simulink model "RPI1Deployment"  (R2026a)
settings: Solver=FixedStepDiscrete  StopTime=inf  FixedStep=rccar.SampleTime  EnableMultiTasking=on
InitFcn:
  | rccarRoot=fileparts(fileparts(fileparts(get_param(bdroot,'FileName')))); addpath(genpath(rccarRoot)); setupRCCarProject; clear rccarRoot;
undefined symbols (not defined in the file): rccar
libraries: raspberrypiNetworklib x3, simulink x1
settings Model: Creator=taegon  LastModifiedBy=taegon
settings SolverCC: PositivePriorityOrder=on
settings OptimizationCC: MaxStackSize=200000
settings HardwareCC: ProdBitPerLong=64.0  ProdLargestAtomicInteger=LongLong  ProdLargestAtomicFloat=Double  ProdHWDeviceType=ARM Compatible->ARM Cortex-A (64-bit)
settings RTWCC: SystemTargetFile=ert.tlc  HardwareBoard=Raspberry Pi (64bit)  TLCOptions="-aInlineSetEventsForThisBaseRateFcn=TLC_FALSE -aSuppressMultiTaskScheduler=TLC_FALSE  -aRateBasedStepFcn=0"  Toolchain=GNU GCC RPIUtils  BuildConfiguration=Faster Runs  Description=Embedded Coder
settings ERTTargetCC: ExtModeTransport=2.0  SupportVariableSizeSignals=on

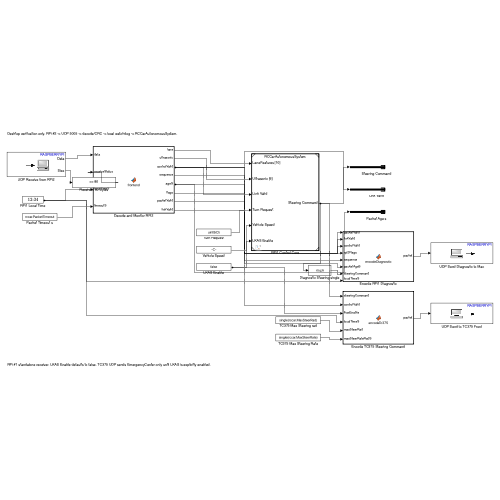
[thumbnail: Simulink's stored preview of the top-level diagram]
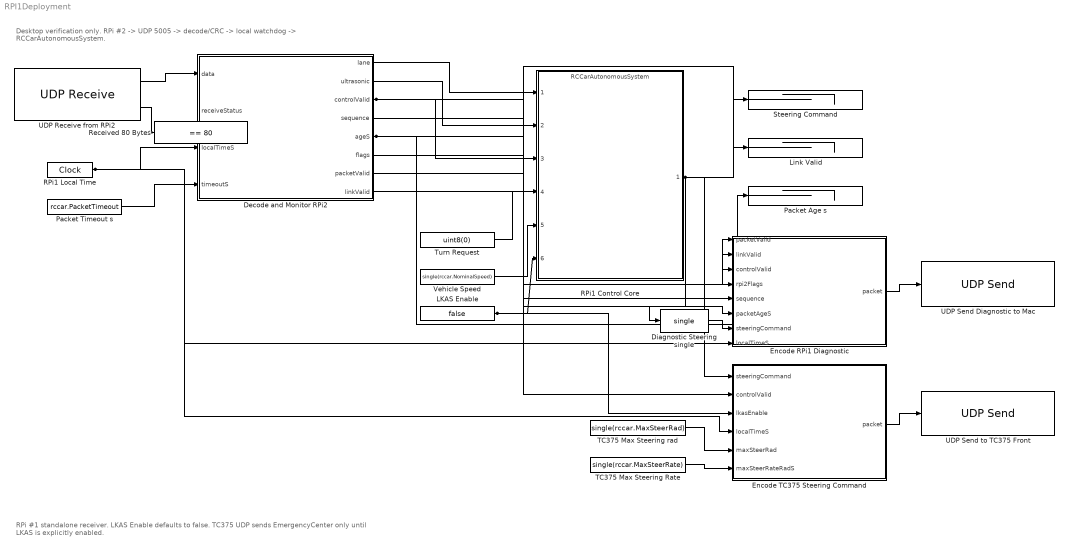
== system RPI1Deployment ==
  note: Desktop verification only. RPi #2 -> UDP 5005 -> decode/CRC -> local watchdog -> RCCarAutonomousSystem.
  note: RPi #1 standalone receiver. LKAS Enable defaults to false. TC375 UDP sends EmergencyCenter only until LKAS is explicitly enabled.
  Decode and Monitor RPi2 : MATLAB Function  TreatAsAtomicUnit=on
  Diagnostic Steering single : DataTypeConversion  OutDataTypeStr=single  SaturateOnIntegerOverflow=off  RndMeth=Floor
  Encode RPi1 Diagnostic : MATLAB Function  TreatAsAtomicUnit=on
  Encode TC375 Steering Command : MATLAB Function  TreatAsAtomicUnit=on
  LKAS Enable : Constant  Value=false  OutDataTypeStr=boolean
  Link Valid : Terminator
  Packet Age s : Terminator
  Packet Timeout s : Constant  Value=rccar.PacketTimeout  OutDataTypeStr=double
  RPi1 Control Core : ModelReference  ModelNameDialog=RCCarAutonomousSystem  SimulationMode=Normal  ModelReferenceVersion=1.3
  RPi1 Local Time : DigitalClock  SampleTime=rccar.SampleTime
  Received 80 Bytes : simulink/Logic and Bit Operations/Compare To Constant  relop===  const=80  OutDataTypeStr=boolean
  Steering Command : Terminator
  TC375 Max Steering Rate : Constant  Value=single(rccar.MaxSteerRate)  OutDataTypeStr=single
  TC375 Max Steering rad : Constant  Value=single(rccar.MaxSteerRad)  OutDataTypeStr=single
  Turn Request : Constant  Value=uint8(0)  OutDataTypeStr=uint8
  UDP Receive from RPi2 : raspberrypiNetworklib/UDP Receive  localURL='0.0.0.0'  localPort=5005  remoteURL='0.0.0.0'  remotePort=-1  recvBufferSize=8192  signalDatatype=uint8  dims=80  isVarSize=off  showBlockingTime=off  blockingTime=0  sampletime=rccar.SampleTime  blockPlatform=Raspberry Pi
  UDP Send Diagnostic to Mac : raspberrypiNetworklib/UDP Send  remoteURL='192.168.201.118'  remotePort=5010  localURL='0.0.0.0'  localPortSource=Automatically determine  localPort=-1  sampletime=rccar.SampleTime  blockPlatform=Raspberry Pi  separateLengthPort=0
  UDP Send to TC375 Front : raspberrypiNetworklib/UDP Send  remoteURL='192.168.10.11'  remotePort=5100  localURL='0.0.0.0'  localPortSource=Specify via dialog  localPort=5101  sampletime=rccar.SampleTime  blockPlatform=Raspberry Pi  separateLengthPort=0
  Vehicle Speed : Constant  Value=single(rccar.NominalSpeed)  OutDataTypeStr=single
  wires:
  RPi1 Local Time/1 -> Decode and Monitor RPi2/3(localTimeS), Encode TC375 Steering Command/4(localTimeS), Encode RPi1 Diagnostic/8(localTimeS)
  Packet Timeout s/1 -> Decode and Monitor RPi2/4(timeoutS)
  Decode and Monitor RPi2/1(lane) -> RPi1 Control Core/1
  Decode and Monitor RPi2/2(ultrasonic) -> RPi1 Control Core/2
  Decode and Monitor RPi2/3(controlValid) -> RPi1 Control Core/3, Link Valid/1, Encode TC375 Steering Command/2(controlValid), Encode RPi1 Diagnostic/3(controlValid)
  Turn Request/1 -> RPi1 Control Core/4
  Vehicle Speed/1 -> RPi1 Control Core/5
  LKAS Enable/1 -> RPi1 Control Core/6, Encode TC375 Steering Command/3(lkasEnable)
  UDP Receive from RPi2/1 -> Decode and Monitor RPi2/1(data)
  UDP Receive from RPi2/2 -> Received 80 Bytes/1
  Received 80 Bytes/1 -> Decode and Monitor RPi2/2(receiveStatus)
  RPi1 Control Core/1 -> Steering Command/1, Encode TC375 Steering Command/1(steeringCommand), Diagnostic Steering single/1
  Decode and Monitor RPi2/5(ageS) -> Packet Age s/1, Encode RPi1 Diagnostic/6(packetAgeS)
  TC375 Max Steering rad/1 -> Encode TC375 Steering Command/5(maxSteerRad)
  TC375 Max Steering Rate/1 -> Encode TC375 Steering Command/6(maxSteerRateRadS)
  Encode TC375 Steering Command/1(packet) -> UDP Send to TC375 Front/1
  Decode and Monitor RPi2/7(packetValid) -> Encode RPi1 Diagnostic/1(packetValid)
  Decode and Monitor RPi2/8(linkValid) -> Encode RPi1 Diagnostic/2(linkValid)
  Decode and Monitor RPi2/6(flags) -> Encode RPi1 Diagnostic/4(rpi2Flags)
  Decode and Monitor RPi2/4(sequence) -> Encode RPi1 Diagnostic/5(sequence)
  Diagnostic Steering single/1 -> Encode RPi1 Diagnostic/7(steeringCommand)
  Encode RPi1 Diagnostic/1(packet) -> UDP Send Diagnostic to Mac/1

== matlab function RPI1Deployment/Encode TC375 Steering Command ==
  data: steeringCommand input single size=1; packet output uint8 size=[40 1]; controlValid input boolean size=1; lkasEnable input boolean size=1; localTimeS input double size=1; maxSteerRad input single size=1; maxSteerRateRadS input single size=1
function packet = encodeTc375(steeringCommand, controlValid, lkasEnable, localTimeS, maxSteerRad, maxSteerRateRadS)
%#codegen
persistent sequence aliveCount
if isempty(sequence), sequence=uint32(0); aliveCount=uint16(0); end
steeringValid=controlValid && lkasEnable && isfinite(steeringCommand) && abs(steeringCommand)<=maxSteerRad;
if steeringValid, safeAngle=steeringCommand; else, safeAngle=single(0); end
emergencyCenter=~steeringValid; controlMode=uint8(steeringValid);
flags=uint8(steeringValid)+bitshift(uint8(emergencyCenter),1)+bitshift(uint8(controlValid),2);
timestampUs=uint64(max(localTimeS,0.0)*1.0e6);
packet=tc375EncodeSteeringPacket(sequence,timestampUs,safeAngle,maxSteerRateRadS,controlMode,flags,aliveCount);
sequence=sequence+uint32(1); aliveCount=aliveCount+uint16(1);
end

== matlab function RPI1Deployment/Decode and Monitor RPi2 ==
  data: data input uint8 size=[80 1]; lane output single size=[10 1]; receiveStatus input boolean size=1; localTimeS input double size=1; timeoutS input double size=1; ultrasonic output single size=[6 1]; controlValid output boolean size=1; sequence output uint32 size=1; ageS output double size=1; flags output uint8 size=1; packetValid output boolean size=1; linkValid output boolean size=1
function [lane, ultrasonic, controlValid, sequence, ageS, flags, packetValid, linkValid] = frontend(data, receiveStatus, localTimeS, timeoutS)
%#codegen
persistent heldLane heldSide heldFlags heldSequence
if isempty(heldLane)
 heldLane=zeros(10,1,'single'); heldSide=single([NaN;NaN]);
 heldFlags=uint8(0); heldSequence=uint32(0);
end
[newLane,newSide,newFlags,newSequence,~,~,packetValid]=rpi2DecodePacket(data,receiveStatus);
if packetValid
 heldLane=newLane; heldSide=newSide; heldFlags=newFlags; heldSequence=newSequence;
end
[linkValid,ageS,~]=rpi2LinkMonitor(localTimeS,packetValid,newSequence,timeoutS,false);
cameraValid=bitand(heldFlags,uint8(1))~=0; laneValid=bitand(heldFlags,uint8(2))~=0;
controlValid=linkValid && cameraValid && laneValid;
lane=heldLane; ultrasonic=single([NaN;NaN;heldSide(1);heldSide(2);NaN;NaN]);
sequence=heldSequence; flags=heldFlags;
end

== matlab function RPI1Deployment/Encode RPi1 Diagnostic ==
  data: packetValid input boolean size=1; packet output uint8 size=[40 1]; linkValid input boolean size=1; controlValid input boolean size=1; rpi2Flags input uint8 size=1; sequence input uint32 size=1; packetAgeS input double size=1; steeringCommand input single size=1; localTimeS input double size=1
function packet = encodeDiagnostic(packetValid, linkValid, controlValid, rpi2Flags, sequence, packetAgeS, steeringCommand, localTimeS)
%#codegen
packet=zeros(40,1,'uint8');
packet(1:4)=uint8([82;49;68;71]); packet(5)=uint8(1);
status=uint8(packetValid)+bitshift(uint8(linkValid),1)+bitshift(uint8(controlValid),2);
packet(6)=status; packet(7)=rpi2Flags; packet(8)=uint8(0);
for k=0:3, packet(9+k)=uint8(bitand(bitshift(sequence,-8*k),uint32(255))); end
ageBytes=typecast(double(packetAgeS),'uint8'); packet(13:20)=ageBytes(:);
steerBytes=typecast(single(steeringCommand),'uint8'); packet(21:24)=steerBytes(:);
timeBytes=typecast(double(localTimeS),'uint8'); packet(25:32)=timeBytes(:);
packet(33:36)=uint8(0); crc=uint32(hex2dec('FFFFFFFF'));
poly=uint32(hex2dec('EDB88320'));
for k=1:36
 crc=bitxor(crc,uint32(packet(k)));
 for bit=1:8
  if bitand(crc,uint32(1))~=0, crc=bitxor(bitshift(crc,-1),poly); else, crc=bitshift(crc,-1); end
 end
end
crc=bitcmp(crc); for k=0:3, packet(37+k)=uint8(bitand(bitshift(crc,-8*k),uint32(255))); end
end
